simulink model "kamyon_model"  (Simulink 7.6)
settings: Solver=ode45  StartTime=0.0  StopTime=80  FixedStep=0.00007  RelTol=1e-3
values from neighbouring files (symbols this model uses):
  ck1 = 10385    [truck.m]    (also in truck_sis.m)
  ck2 = 10385    [truck.m]    (also in truck_sis.m)
  ck3 = 14432    [truck.m]    (also in truck_sis.m)
  ck4 = 10385    [truck.m]    (also in truck_sis.m)
  ck5 = 10385    [truck.m]    (also in truck_sis.m)
  ck6 = 14432    [truck.m]    (also in truck_sis.m)
  dyk = 0.007    [truck.m]    (also in truck_sis.m)
  kk1 = 108000    [truck.m]    (also in truck_sis.m)
  kk10 = 1057170    [truck.m]    (also in truck_sis.m)
  kk11 = 155500    [truck.m]    (also in truck_sis.m)
  kk12 = 2057694    [truck.m]    (also in truck_sis.m)
  kk2 = 944046    [truck.m]    (also in truck_sis.m)
  kk3 = 230000    [truck.m]    (also in truck_sis.m)
  kk4 = 1057170    [truck.m]    (also in truck_sis.m)
  kk5 = 155500    [truck.m]    (also in truck_sis.m)
  kk6 = 2057694    [truck.m]    (also in truck_sis.m)
  kk7 = 108000    [truck.m]    (also in truck_sis.m)
  kk8 = 944046    [truck.m]    (also in truck_sis.m)
  kk9 = 230000    [truck.m]    (also in truck_sis.m)
  Lk1 = 3.812    [truck.m]    (also in truck_sis.m)
  Lk2 = 5.042    [truck.m]    (also in truck_sis.m)
  Lk3 = 0.84    [truck.m]    (also in truck_sis.m)
  Lk4 = 1.2    [truck.m]    (also in truck_sis.m)
  Lk5 = 1.2    [truck.m]    (also in truck_sis.m)
  mk2 = 375    [truck.m]    (also in truck_sis.m)
  mk3 = 400    [truck.m]    (also in truck_sis.m)
  mk4 = 730    [truck.m]    (also in truck_sis.m)
  mk5 = 375    [truck.m]    (also in truck_sis.m)
  mk6 = 400    [truck.m]    (also in truck_sis.m)
  mk7 = 730    [truck.m]    (also in truck_sis.m)
  Vk = 25    [truck.m]    (also in truck_sis.m = 16.6666666667)
  wk = Vk/dyk    (= 3571.42857143)    [truck.m]    (also in truck_sis.m = 2380.95238095)
settings Model: Creator=aster  LastModifiedBy=user
settings SolverCC: NumberNewtonIterations=100  ZeroCrossAlgorithm=Adaptive
settings OptimizationCC: InitFltsAndDblsToZero=on
settings DebuggingCC: StrictBusMsg=Warning

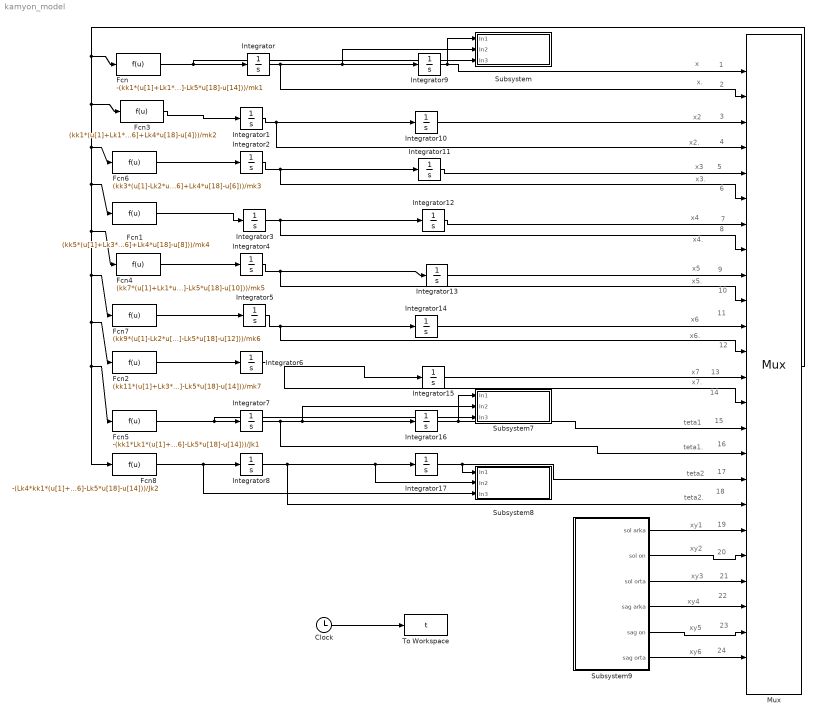
== system kamyon_model ==
  note: x
  note: x.
  note: x2
  note: x2.
  note: x3
  note: x3.
  note: x4
  note: x4.
  note: x5
  note: x5.
  note: x6
  note: x6.
  note: x7
  note: x7.
  note: teta1
  note: teta1.
  note: teta2
  note: teta2.
  note: xy1
  note: xy2
  note: xy3
  note: xy4
  note: xy5
  note: xy6
  note: 1
  note: 2
  note: 3
  note: 4
  note: 5
  note: 6
  note: 7
  note: 8
  note: 9
  note: 10
  note: 11
  note: 12
  note: 13
  note: 14
  note: 15
  note: 16
  note: 17
  note: 18
  note: 19
  note: 20
  note: 21
  note: 22
  note: 23
  note: 24
  Clock : Clock
      settings: Decimation=10
  Fcn : Fcn  Expr=-(kk1*(u[1]+Lk1*u[15]+Lk4*u[17]-u[3])+kk3*(u[1]-Lk2*u[15]+Lk4*u[17]-u[5])+kk5*(u[1]+Lk3*u[15]+Lk4*u[17]-u[7])+kk7*(u[1]+Lk1*u[15]-Lk5*u[17]-u[9])+kk9*(u[1]-Lk2*u[15]-Lk5*u[17]-u[11])+kk11*(u[1]+Lk3*u[15]-Lk5*u[17]-u[13])+ck1*(u[2]+Lk1*u[16]+Lk4*u[18]-u[4])+ck2*(u[2]-Lk2*u[16]+Lk4*u[18]-u[6])+ck3*(u[2]+Lk3*u[16]+Lk4*u[18]-u[8])+ck4*(u[2]+Lk1*u[16]-Lk5*u[18]-u[10])+ck5*(u[2]-Lk2*u[16]-Lk5*u[18]-u[12])+ck6*(u[2]+Lk3*u[16]-Lk5*u[18]-u[14]))/mk1
  Fcn1 : Fcn  Expr=(kk5*(u[1]+Lk3*u[15]+Lk4*u[17]-u[7])-kk6*(u[7]-u[21])+ck3*(u[2]-Lk3*u[16]+Lk4*u[18]-u[8]))/mk4
  Fcn2 : Fcn  Expr=(kk11*(u[1]+Lk3*u[15]-Lk5*u[17]-u[13])-kk12*(u[13]-u[24])+ck6*(u[2]+Lk3*u[16]-Lk5*u[18]-u[14]))/mk7
  Fcn3 : Fcn  Expr=(kk1*(u[1]+Lk1*u[15]+Lk4*u[17]-u[3])-kk2*(u[3]-u[19])+ck1*(u[2]+Lk1*u[16]+Lk4*u[18]-u[4]))/mk2
  Fcn4 : Fcn  Expr=(kk7*(u[1]+Lk1*u[15]-Lk5*u[17]-u[9])-kk8*(u[9]-u[22])+ck4*(u[2]+Lk1*u[16]-Lk5*u[18]-u[10]))/mk5
  Fcn5 : Fcn  Expr=-(kk1*Lk1*(u[1]+Lk1*u[15]+Lk4*u[17]-u[3])-kk3*Lk2*(u[1]-Lk2*u[15]+Lk4*u[17]-u[5])+kk5*Lk3*(u[1]+Lk3*u[15]+Lk4*u[17]-u[7])+kk7*Lk1*(u[1]+Lk1*u[15]-Lk5*u[17]-u[9])-kk9*Lk2*(u[1]-Lk2*u[15]-Lk5*u[17]-u[11])+kk11*Lk3*(u[1]+Lk3*u[15]-Lk5*u[17]-u[13])+ck1*Lk1*(u[2]+Lk1*u[16]+Lk4*u[18]-u[4])-ck2*Lk2*(u[2]-Lk2*u[16]+Lk4*u[18]-u[6])+ck3*Lk3*(u[2]+Lk3*u[16]+Lk4*u[18]-u[8])+ck4*Lk1*(u[2]+Lk1*u[16]-Lk5*u[18]-u[10])-ck5*Lk2*(u[2]-Lk2*u[16]-Lk5*u[18]-u[12])+ck6*Lk3*(u[2]+Lk3*u[16]-Lk5*u[18]-u[14]))/Jk1
  Fcn6 : Fcn  Expr=(kk3*(u[1]-Lk2*u[15]+Lk4*u[17]-u[5])-kk4*(u[5]-u[20])+ck2*(u[2]-Lk2*u[16]+Lk4*u[18]-u[6]))/mk3
  Fcn7 : Fcn  Expr=(kk9*(u[1]-Lk2*u[15]-Lk5*u[17]-u[11])-kk10*(u[11]-u[23])+ck5*(u[2]-Lk2*u[16]-Lk5*u[18]-u[12]))/mk6
  Fcn8 : Fcn  Expr=-(Lk4*kk1*(u[1]+Lk1*u[15]+Lk4*u[17]-u[3])+Lk4*kk3*(u[1]-Lk2*u[15]+Lk4*u[17]-u[5])+Lk4*kk5*(u[1]+Lk3*u[15]+Lk4*u[17]-u[7])-Lk5*kk7*(u[1]+Lk1*u[15]-Lk5*u[17]-u[9])-Lk5*kk9*(u[1]-Lk2*u[15]-Lk5*u[17]-u[11])-Lk5*kk11*(u[1]+Lk3*u[15]-Lk5*u[17]-u[13])+Lk4*ck1*(u[2]+Lk1*u[16]+Lk4*u[18]-u[4])+Lk4*ck2*(u[2]-Lk2*u[16]+Lk4*u[18]-u[6])+Lk4*ck3*(u[2]+Lk3*u[16]+Lk4*u[18]-u[8])-Lk5*ck4*(u[2]+Lk1*u[16]-Lk5*u[18]-u[10])-Lk5*ck5*(u[2]-Lk2*u[16]-Lk5*u[18]-u[12])-Lk5*ck6*(u[2]+Lk3*u[16]-Lk5*u[18]-u[14]))/Jk2
  Integrator{,1..17} (18 alike) : Integrator
  Mux : Mux  Inputs=24
  Subsystem : Subsystem
  Subsystem7 : Subsystem
  Subsystem8 : Subsystem
  Subsystem9 : Subsystem
  To Workspace : ToWorkspace  VariableName=t  SampleTime=-1  SaveFormat=Array
  wires:
  Fcn/1 -> Integrator/1, Subsystem/3(In3)
  Fcn3/1 -> Integrator1/1
  Fcn6/1 -> Integrator2/1
  Fcn1/1 -> Integrator3/1
  Fcn4/1 -> Integrator4/1
  Fcn7/1 -> Integrator5/1
  Fcn2/1 -> Integrator6/1
  Fcn5/1 -> Integrator7/1, Subsystem7/3(In3)
  Fcn8/1 -> Integrator8/1, Subsystem8/3(In3)
  Integrator/1 -> Mux/2, Integrator9/1, Subsystem/2(In2)
  Integrator1/1 -> Mux/4, Integrator10/1
  Integrator2/1 -> Mux/6, Integrator11/1
  Integrator3/1 -> Mux/8, Integrator12/1
  Integrator4/1 -> Mux/10, Integrator13/1
  Integrator5/1 -> Mux/12, Integrator14/1
  Integrator6/1 -> Mux/14, Integrator15/1
  Integrator7/1 -> Mux/16, Integrator16/1, Subsystem7/2(In2)
  Integrator8/1 -> Mux/18, Integrator17/1, Subsystem8/2(In2)
  Mux/1 -> Fcn8/1, Fcn5/1, Fcn2/1, Fcn7/1, Fcn4/1, Fcn1/1, Fcn6/1, Fcn3/1, Fcn/1
  Integrator9/1 -> Subsystem/1(In1), Mux/1
  Integrator10/1 -> Mux/3
  Integrator11/1 -> Mux/5
  Integrator12/1 -> Mux/7
  Integrator13/1 -> Mux/9
  Integrator14/1 -> Mux/11
  Integrator15/1 -> Mux/13
  Integrator16/1 -> Mux/15, Subsystem7/1(In1)
  Integrator17/1 -> Mux/17, Subsystem8/1(In1)
  Clock/1 -> To Workspace/1
  Subsystem9/1(sol arka) -> Mux/19
  Subsystem9/2(sol on) -> Mux/20
  Subsystem9/3(sol orta) -> Mux/21
  Subsystem9/4(sag arka) -> Mux/22
  Subsystem9/5(sag on) -> Mux/23
  Subsystem9/6(sag orta) -> Mux/24

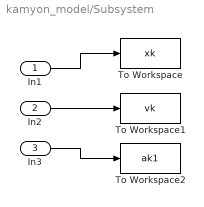
== system kamyon_model/Subsystem ==
  In1 : Inport
  In2 : Inport  Port=2
  In3 : Inport  Port=3
  To Workspace : ToWorkspace  VariableName=xk  SampleTime=-1  SaveFormat=Array
  To Workspace1 : ToWorkspace  VariableName=vk  SampleTime=-1  SaveFormat=Array
  To Workspace2 : ToWorkspace  VariableName=ak1  SampleTime=-1  SaveFormat=Array
  wires:
  In1/1 -> To Workspace/1
  In2/1 -> To Workspace1/1
  In3/1 -> To Workspace2/1

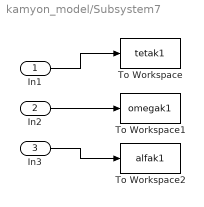
== system kamyon_model/Subsystem7 ==
  In1 : Inport
  In2 : Inport  Port=2
  In3 : Inport  Port=3
  To Workspace : ToWorkspace  VariableName=tetak1  SampleTime=-1  SaveFormat=Array
  To Workspace1 : ToWorkspace  VariableName=omegak1  SampleTime=-1  SaveFormat=Array
  To Workspace2 : ToWorkspace  VariableName=alfak1  SampleTime=-1  SaveFormat=Array
  wires:
  In3/1 -> To Workspace2/1
  In2/1 -> To Workspace1/1
  In1/1 -> To Workspace/1

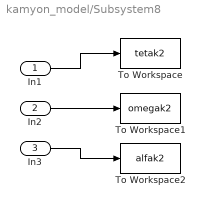
== system kamyon_model/Subsystem8 ==
  In1 : Inport
  In2 : Inport  Port=2
  In3 : Inport  Port=3
  To Workspace : ToWorkspace  VariableName=tetak2  SampleTime=-1  SaveFormat=Array
  To Workspace1 : ToWorkspace  VariableName=omegak2  SampleTime=-1  SaveFormat=Array
  To Workspace2 : ToWorkspace  VariableName=alfak2  SampleTime=-1  SaveFormat=Array
  wires:
  In1/1 -> To Workspace/1
  In2/1 -> To Workspace1/1
  In3/1 -> To Workspace2/1

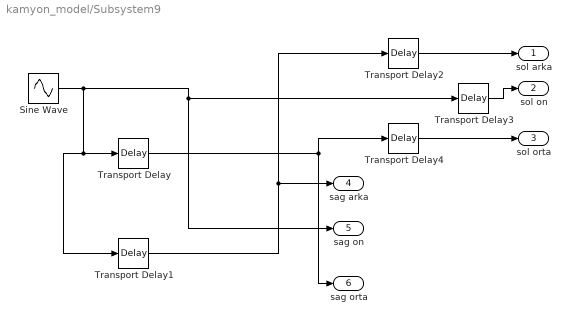
== system kamyon_model/Subsystem9 ==
  Sine Wave : Sin  Amplitude=dyk  Frequency=wk  SampleTime=0
  Transport Delay : TransportDelay  DelayTime=(Lk2+Lk3)/Vk
  Transport Delay1 : TransportDelay  DelayTime=(Lk1+Lk2)/Vk
  Transport Delay2 : TransportDelay  DelayTime=0.001
  Transport Delay3 : TransportDelay  DelayTime=0.001
  Transport Delay4 : TransportDelay  DelayTime=0.001
  sol arka : Outport
  sol on : Outport  Port=2
  sol orta : Outport  Port=3
  sag arka : Outport  Port=4
  sag on : Outport  Port=5
  sag orta : Outport  Port=6
  wires:
  Sine Wave/1 -> sag on/1, Transport Delay3/1, Transport Delay/1, Transport Delay1/1
  Transport Delay/1 -> sag orta/1, Transport Delay4/1
  Transport Delay1/1 -> sag arka/1, Transport Delay2/1
  Transport Delay2/1 -> sol arka/1
  Transport Delay3/1 -> sol on/1
  Transport Delay4/1 -> sol orta/1
